simulink model "Aero_VarVsp"  (R2016b)
settings: Solver=VariableStepAuto  StartTime=0.0  StopTime=10.0  RelTol=1e-3
undefined symbols (not defined in the file or in its folder): AC
libraries: OpenFlightUtilLib x3
settings Model: Creator=UAVLAB  LastModifiedBy=rega0051
settings DataIOCC: ExternalInput=simIn  InitialState=simStateInit  StateSaveName=simStates  TimeSaveName=simTime  OutputSaveName=simOut  SignalLoggingName=simLog  DSMLoggingName=simData

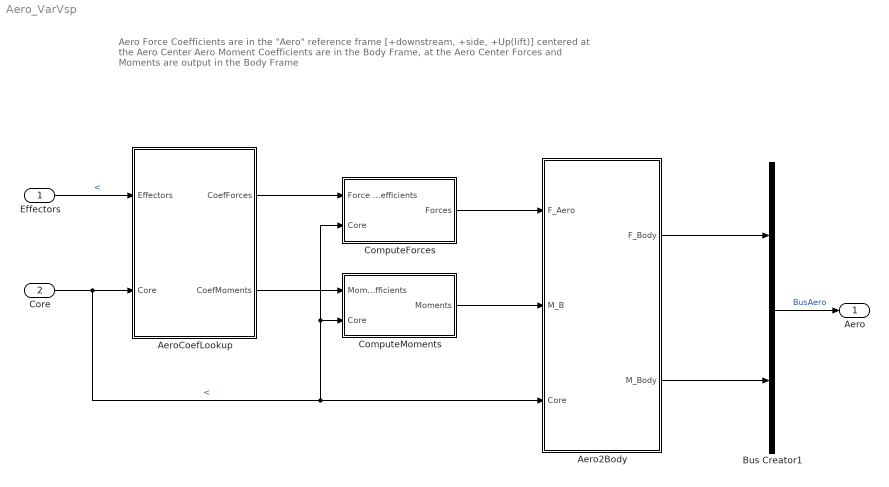
== system Aero_VarVsp ==
  note: Aero Force Coefficients are in the "Aero" reference frame [+downstream, +side, +Up(lift)] centered at the Aero Center
      | Aero Moment Coefficients are in the Body Frame, at the Aero Center
      |
      | Forces and Moments are output in the Body Frame
  Effectors : Inport  OutDataTypeStr=Bus: BusEff
  Core : Inport  Port=2  OutDataTypeStr=Bus: BusCore
  Aero2Body : Subsystem
  AeroCoefLookup : Subsystem
  Bus Creator1 : BusCreator  Inputs=2  OutDataTypeStr=Bus: BusAero
      settings: AttributesFormatString=%<OutDataTypeStr>
  ComputeForces : Subsystem
  ComputeMoments : Subsystem
  Aero : Outport  OutDataTypeStr=Bus: BusAero
  wires:
  Effectors/1 -> AeroCoefLookup/1(Effectors)  "<"
  ComputeForces/1(Forces) -> Aero2Body/1(F_Aero)
  ComputeMoments/1(Moments) -> Aero2Body/2(M_B)
  Aero2Body/1(F_Body) -> Bus Creator1/1
  Aero2Body/2(M_Body) -> Bus Creator1/2
  AeroCoefLookup/1(CoefForces) -> ComputeForces/1(Force Coefficients)
  AeroCoefLookup/2(CoefMoments) -> ComputeMoments/1(Moment Coefficients)
  Bus Creator1/1 -> Aero/1  "BusAero"
  Core/1 -> ComputeForces/2(Core), ComputeMoments/2(Core), Aero2Body/3(Core), AeroCoefLookup/2(Core)  "<"

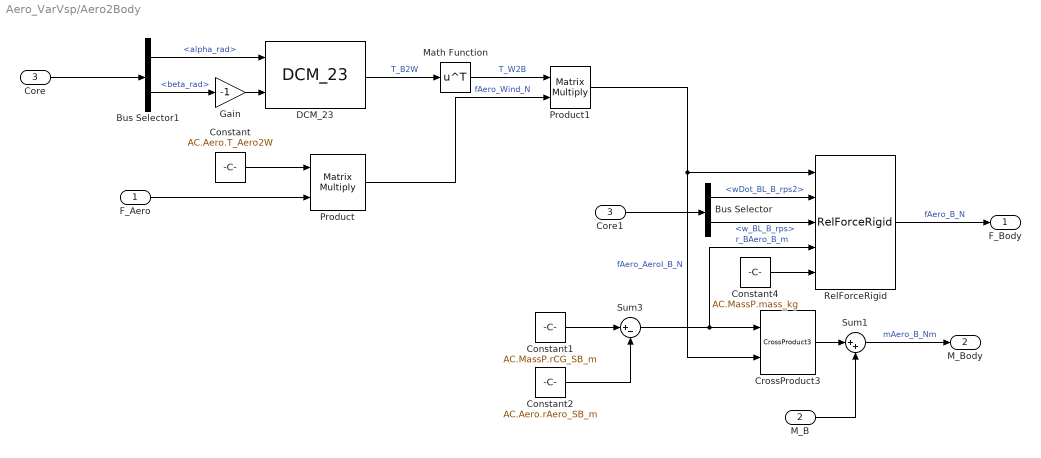
== system Aero_VarVsp/Aero2Body ==
  F_Aero : Inport
  M_B : Inport  Port=2
  Core : Inport  Port=3
  Bus Selector : BusSelector  OutputSignals=BusEom.wDot_BL_B_rps2,BusEom.w_BL_B_rps
  Bus Selector1 : BusSelector  OutputSignals=BusAux.BusFlow.alpha_rad,BusAux.BusFlow.beta_rad
  Constant : Constant  Value=AC.Aero.T_Aero2W
      settings: AttributesFormatString=%<Value>
  Constant1 : Constant  Value=AC.MassP.rCG_SB_m
      settings: AttributesFormatString=%<Value>
  Constant2 : Constant  Value=AC.Aero.rAero_SB_m
      settings: AttributesFormatString=%<Value>
  Constant4 : Constant  Value=AC.MassP.mass_kg
      settings: AttributesFormatString=%<Value>
  Core1 : InportShadow  Port=3
  CrossProduct3 : OpenFlightUtilLib/Math/CrossProduct3
  DCM_23 : OpenFlightUtilLib/Transformations/DCM_23
  Gain : Gain  Gain=-1
  Math Function : Math  Operator=transpose  SaturateOnIntegerOverflow=on
  Product : Product  Multiplication=Matrix(*)  RndMeth=Zero
  Product1 : Product  Multiplication=Matrix(*)  RndMeth=Zero
  RelForceRigid : OpenFlightUtilLib/Kinematics and Dynamics/RelForceRigid
  Sum1 : Sum  Inputs=|++  SaturateOnIntegerOverflow=on
  Sum3 : Sum  Inputs=|+-  SaturateOnIntegerOverflow=on
  F_Body : Outport
  M_Body : Outport  Port=2
  wires:
  Constant1/1 -> Sum3/1
  Constant2/1 -> Sum3/2
  Bus Selector/1 -> RelForceRigid/2  "<wDot_BL_B_rps2>"
  Bus Selector/2 -> RelForceRigid/3  "<w_BL_B_rps>"
  F_Aero/1 -> Product/2
  Constant/1 -> Product/1
  Core/1 -> Bus Selector1/1
  Math Function/1 -> Product1/1  "T_W2B"
  DCM_23/1 -> Math Function/1  "T_B2W"
  Product/1 -> Product1/2  "fAero_Wind_N"
  Product1/1 -> CrossProduct3/2, RelForceRigid/1  "fAero_AeroI_B_N"
  Sum3/1 -> RelForceRigid/4, CrossProduct3/1  "r_BAero_B_m"
  Core1/1 -> Bus Selector/1
  RelForceRigid/1 -> F_Body/1  "fAero_B_N"
  M_B/1 -> Sum1/2
  CrossProduct3/1 -> Sum1/1
  Sum1/1 -> M_Body/1  "mAero_B_Nm"
  Constant4/1 -> RelForceRigid/5
  Bus Selector1/1 -> DCM_23/1  "<alpha_rad>"
  Bus Selector1/2 -> Gain/1  "<beta_rad>"
  Gain/1 -> DCM_23/2

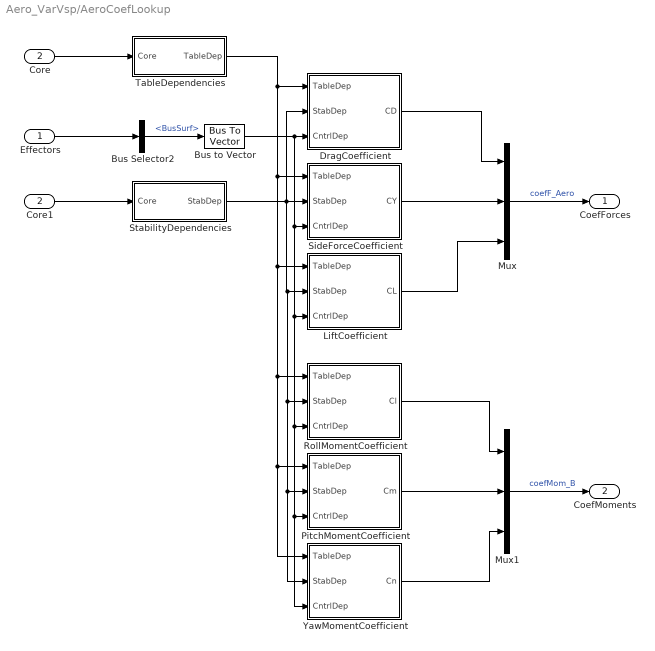
== system Aero_VarVsp/AeroCoefLookup ==
  Effectors : Inport
  Core : Inport  Port=2
  Bus Selector2 : BusSelector  OutputSignals=BusSurf
  Bus to Vector : BusToVector
  Core1 : InportShadow  Port=2
  DragCoefficient : Subsystem
  LiftCoefficient : Subsystem
  Mux : Mux  Inputs=3
  Mux1 : Mux  Inputs=3
  PitchMomentCoefficient : Subsystem
  RollMomentCoefficient : Subsystem
  SideForceCoefficient : Subsystem
  StabilityDependencies : Subsystem
  TableDependencies : Subsystem
  YawMomentCoefficient : Subsystem
  CoefForces : Outport
  CoefMoments : Outport  Port=2
  wires:
  Mux1/1 -> CoefMoments/1  "coefMom_B"
  SideForceCoefficient/1(CY) -> Mux/2
  PitchMomentCoefficient/1(Cm) -> Mux1/2
  Mux/1 -> CoefForces/1  "coefF_Aero"
  RollMomentCoefficient/1(Cl) -> Mux1/1
  LiftCoefficient/1(CL) -> Mux/3
  YawMomentCoefficient/1(Cn) -> Mux1/3
  DragCoefficient/1(CD) -> Mux/1
  Bus Selector2/1 -> Bus to Vector/1  "<BusSurf>"
  TableDependencies/1(TableDep) -> DragCoefficient/1(TableDep), SideForceCoefficient/1(TableDep), YawMomentCoefficient/1(TableDep), PitchMomentCoefficient/1(TableDep), RollMomentCoefficient/1(TableDep), LiftCoefficient/1(TableDep)
  Effectors/1 -> Bus Selector2/1
  Core1/1 -> StabilityDependencies/1(Core)
  StabilityDependencies/1(StabDep) -> DragCoefficient/2(StabDep), YawMomentCoefficient/2(StabDep), PitchMomentCoefficient/2(StabDep), RollMomentCoefficient/2(StabDep), LiftCoefficient/2(StabDep), SideForceCoefficient/2(StabDep)
  Bus to Vector/1 -> DragCoefficient/3(CntrlDep), YawMomentCoefficient/3(CntrlDep), PitchMomentCoefficient/3(CntrlDep), RollMomentCoefficient/3(CntrlDep), LiftCoefficient/3(CntrlDep), SideForceCoefficient/3(CntrlDep)
  Core/1 -> TableDependencies/1(Core)

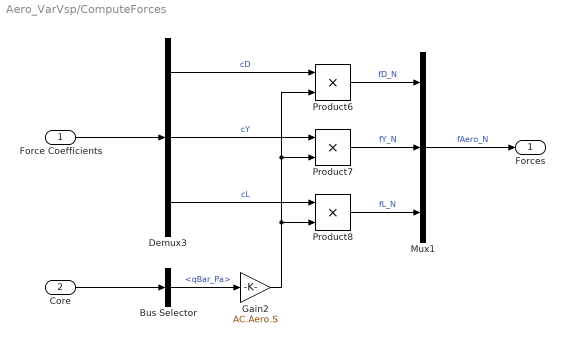
== system Aero_VarVsp/ComputeForces ==
  Force Coefficients : Inport
  Core : Inport  Port=2
  Bus Selector : BusSelector  OutputSignals=BusAux.BusFlow.qBar_Pa
  Demux3 : Demux  Outputs=3
  Gain2 : Gain  Gain=AC.Aero.S  SaturateOnIntegerOverflow=on  OutDataTypeStr=Inherit: Same as input  ParamDataTypeStr=Inherit: Same as input
      settings: AttributesFormatString=%<Gain>
  Mux1 : Mux  Inputs=3
  Product6 : Product  SaturateOnIntegerOverflow=on  InputSameDT=on  OutDataTypeStr=Inherit: Same as first input
  Product7 : Product  SaturateOnIntegerOverflow=on  InputSameDT=on  OutDataTypeStr=Inherit: Same as first input
  Product8 : Product  SaturateOnIntegerOverflow=on  InputSameDT=on  OutDataTypeStr=Inherit: Same as first input
  Forces : Outport
  wires:
  Product6/1 -> Mux1/1  "fD_N"
  Product8/1 -> Mux1/3  "fL_N"
  Product7/1 -> Mux1/2  "fY_N"
  Mux1/1 -> Forces/1  "fAero_N"
  Demux3/2 -> Product7/1  "cY"
  Demux3/1 -> Product6/1  "cD"
  Demux3/3 -> Product8/1  "cL"
  Force Coefficients/1 -> Demux3/1
  Gain2/1 -> Product6/2, Product7/2, Product8/2
  Bus Selector/1 -> Gain2/1  "<qBar_Pa>"
  Core/1 -> Bus Selector/1

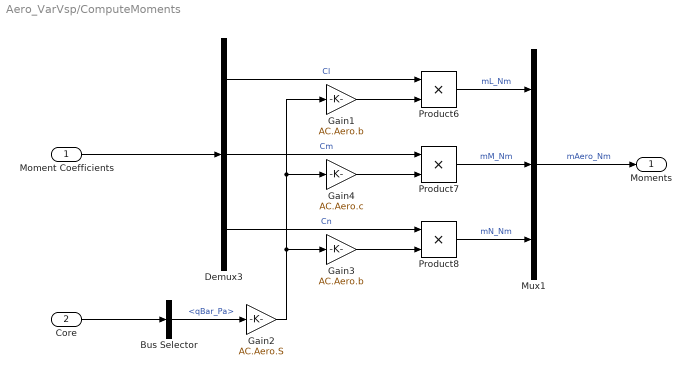
== system Aero_VarVsp/ComputeMoments ==
  Moment Coefficients : Inport
  Core : Inport  Port=2
  Bus Selector : BusSelector  OutputSignals=BusAux.BusFlow.qBar_Pa
  Demux3 : Demux  Outputs=3
  Gain1 : Gain  Gain=AC.Aero.b  SaturateOnIntegerOverflow=on  OutDataTypeStr=Inherit: Same as input  ParamDataTypeStr=Inherit: Same as input
      settings: AttributesFormatString=%<Gain>
  Gain2 : Gain  Gain=AC.Aero.S  SaturateOnIntegerOverflow=on  OutDataTypeStr=Inherit: Same as input  ParamDataTypeStr=Inherit: Same as input
      settings: AttributesFormatString=%<Gain>
  Gain3 : Gain  Gain=AC.Aero.b  SaturateOnIntegerOverflow=on  OutDataTypeStr=Inherit: Same as input  ParamDataTypeStr=Inherit: Same as input
      settings: AttributesFormatString=%<Gain>
  Gain4 : Gain  Gain=AC.Aero.c  SaturateOnIntegerOverflow=on  OutDataTypeStr=Inherit: Same as input  ParamDataTypeStr=Inherit: Same as input
      settings: AttributesFormatString=%<Gain>
  Mux1 : Mux  Inputs=3
  Product6 : Product  SaturateOnIntegerOverflow=on  InputSameDT=on  OutDataTypeStr=Inherit: Same as first input
  Product7 : Product  SaturateOnIntegerOverflow=on  InputSameDT=on  OutDataTypeStr=Inherit: Same as first input
  Product8 : Product  SaturateOnIntegerOverflow=on  InputSameDT=on  OutDataTypeStr=Inherit: Same as first input
  Moments : Outport
  wires:
  Product6/1 -> Mux1/1  "mL_Nm"
  Product8/1 -> Mux1/3  "mN_Nm"
  Moment Coefficients/1 -> Demux3/1
  Product7/1 -> Mux1/2  "mM_Nm"
  Gain3/1 -> Product8/2
  Mux1/1 -> Moments/1  "mAero_Nm"
  Gain1/1 -> Product6/2
  Gain2/1 -> Gain1/1, Gain4/1, Gain3/1
  Demux3/2 -> Product7/1  "Cm"
  Gain4/1 -> Product7/2
  Demux3/1 -> Product6/1  "Cl"
  Demux3/3 -> Product8/1  "Cn"
  Bus Selector/1 -> Gain2/1  "<qBar_Pa>"
  Core/1 -> Bus Selector/1

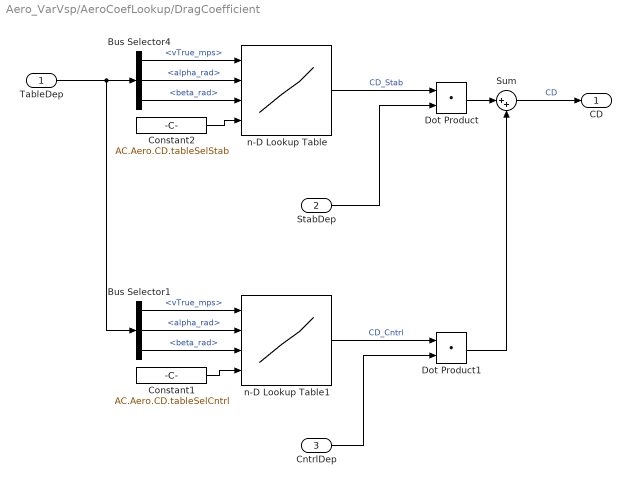
== system Aero_VarVsp/AeroCoefLookup/DragCoefficient ==
  TableDep : Inport
  StabDep : Inport  Port=2
  CntrlDep : Inport  Port=3
  Bus Selector1 : BusSelector  OutputSignals=vTrue_mps,alpha_rad,beta_rad
  Bus Selector4 : BusSelector  OutputSignals=vTrue_mps,alpha_rad,beta_rad
  Constant1 : Constant  Value=AC.Aero.CD.tableSelCntrl
      settings: AttributesFormatString=%<Value>
  Constant2 : Constant  Value=AC.Aero.CD.tableSelStab
      settings: AttributesFormatString=%<Value>
  Dot Product : DotProduct  InputSameDT=on  OutDataTypeStr=Inherit: Inherit via internal rule
  Dot Product1 : DotProduct  InputSameDT=on  OutDataTypeStr=Inherit: Inherit via internal rule
  Sum : Sum  Inputs=|++
  n-D Lookup Table : Lookup_n-D  NumberOfTableDimensions=AC.Aero.tableDim  BreakpointsForDimension1=AC.Aero.breakPts{1}  BreakpointsForDimension2=AC.Aero.breakPts{2}  BreakpointsForDimension3=AC.Aero.breakPts{3}  BreakpointsForDimension4=AC.Aero.CD.tableSelStab  Table=AC.Aero.CD.tableStab  InternalRulePriority=Speed  RndMeth=Simplest  InputSameDT=on
      settings: AttributesFormatString=%<Table>
  n-D Lookup Table1 : Lookup_n-D  NumberOfTableDimensions=AC.Aero.tableDim  BreakpointsForDimension1=AC.Aero.breakPts{1}  BreakpointsForDimension2=AC.Aero.breakPts{2}  BreakpointsForDimension3=AC.Aero.breakPts{3}  BreakpointsForDimension4=AC.Aero.CD.tableSelCntrl  Table=AC.Aero.CD.tableCntrl  InternalRulePriority=Speed  RndMeth=Simplest  InputSameDT=on
      settings: AttributesFormatString=%<Table>
  CD : Outport
  wires:
  Dot Product/1 -> Sum/1
  Bus Selector4/1 -> n-D Lookup Table/1  "<vTrue_mps>"
  Bus Selector4/2 -> n-D Lookup Table/2  "<alpha_rad>"
  Constant2/1 -> n-D Lookup Table/4
  n-D Lookup Table/1 -> Dot Product/1  "CD_Stab"
  StabDep/1 -> Dot Product/2
  TableDep/1 -> Bus Selector1/1, Bus Selector4/1
  Constant1/1 -> n-D Lookup Table1/4
  CntrlDep/1 -> Dot Product1/2
  n-D Lookup Table1/1 -> Dot Product1/1  "CD_Cntrl"
  Dot Product1/1 -> Sum/2
  Sum/1 -> CD/1  "CD"
  Bus Selector4/3 -> n-D Lookup Table/3  "<beta_rad>"
  Bus Selector1/1 -> n-D Lookup Table1/1  "<vTrue_mps>"
  Bus Selector1/2 -> n-D Lookup Table1/2  "<alpha_rad>"
  Bus Selector1/3 -> n-D Lookup Table1/3  "<beta_rad>"

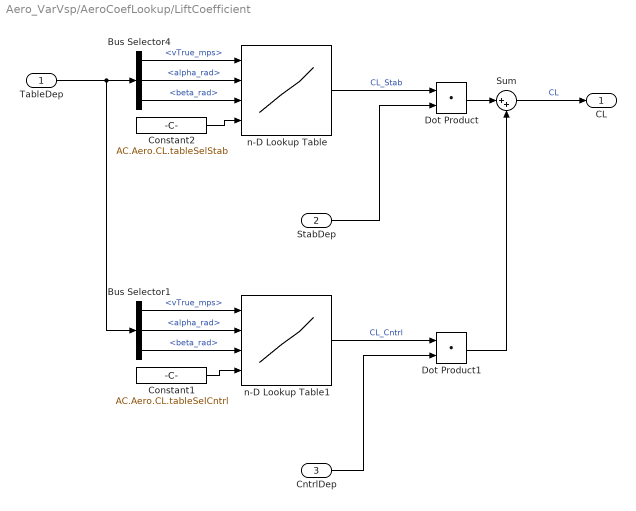
== system Aero_VarVsp/AeroCoefLookup/LiftCoefficient ==
  TableDep : Inport
  StabDep : Inport  Port=2
  CntrlDep : Inport  Port=3
  Bus Selector1 : BusSelector  OutputSignals=vTrue_mps,alpha_rad,beta_rad
  Bus Selector4 : BusSelector  OutputSignals=vTrue_mps,alpha_rad,beta_rad
  Constant1 : Constant  Value=AC.Aero.CL.tableSelCntrl
      settings: AttributesFormatString=%<Value>
  Constant2 : Constant  Value=AC.Aero.CL.tableSelStab
      settings: AttributesFormatString=%<Value>
  Dot Product : DotProduct  InputSameDT=on  OutDataTypeStr=Inherit: Inherit via internal rule
  Dot Product1 : DotProduct  InputSameDT=on  OutDataTypeStr=Inherit: Inherit via internal rule
  Sum : Sum  Inputs=|++
  n-D Lookup Table : Lookup_n-D  NumberOfTableDimensions=AC.Aero.tableDim  BreakpointsForDimension1=AC.Aero.breakPts{1}  BreakpointsForDimension2=AC.Aero.breakPts{2}  BreakpointsForDimension3=AC.Aero.breakPts{3}  BreakpointsForDimension4=AC.Aero.CL.tableSelStab  Table=AC.Aero.CL.tableStab  InternalRulePriority=Speed  RndMeth=Simplest  InputSameDT=on
      settings: AttributesFormatString=%<Table>
  n-D Lookup Table1 : Lookup_n-D  NumberOfTableDimensions=AC.Aero.tableDim  BreakpointsForDimension1=AC.Aero.breakPts{1}  BreakpointsForDimension2=AC.Aero.breakPts{2}  BreakpointsForDimension3=AC.Aero.breakPts{3}  BreakpointsForDimension4=AC.Aero.CL.tableSelCntrl  Table=AC.Aero.CL.tableCntrl  InternalRulePriority=Speed  RndMeth=Simplest  InputSameDT=on
      settings: AttributesFormatString=%<Table>
  CL : Outport
  wires:
  Dot Product/1 -> Sum/1
  Constant2/1 -> n-D Lookup Table/4
  n-D Lookup Table/1 -> Dot Product/1  "CL_Stab"
  StabDep/1 -> Dot Product/2
  TableDep/1 -> Bus Selector1/1, Bus Selector4/1
  Constant1/1 -> n-D Lookup Table1/4
  CntrlDep/1 -> Dot Product1/2
  n-D Lookup Table1/1 -> Dot Product1/1  "CL_Cntrl"
  Dot Product1/1 -> Sum/2
  Sum/1 -> CL/1  "CL"
  Bus Selector4/3 -> n-D Lookup Table/3  "<beta_rad>"
  Bus Selector4/2 -> n-D Lookup Table/2  "<alpha_rad>"
  Bus Selector4/1 -> n-D Lookup Table/1  "<vTrue_mps>"
  Bus Selector1/1 -> n-D Lookup Table1/1  "<vTrue_mps>"
  Bus Selector1/2 -> n-D Lookup Table1/2  "<alpha_rad>"
  Bus Selector1/3 -> n-D Lookup Table1/3  "<beta_rad>"

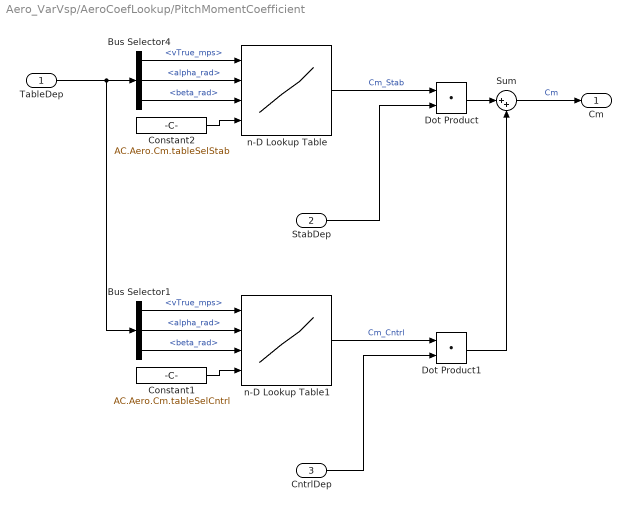
== system Aero_VarVsp/AeroCoefLookup/PitchMomentCoefficient ==
  TableDep : Inport
  StabDep : Inport  Port=2
  CntrlDep : Inport  Port=3
  Bus Selector1 : BusSelector  OutputSignals=vTrue_mps,alpha_rad,beta_rad
  Bus Selector4 : BusSelector  OutputSignals=vTrue_mps,alpha_rad,beta_rad
  Constant1 : Constant  Value=AC.Aero.Cm.tableSelCntrl
      settings: AttributesFormatString=%<Value>
  Constant2 : Constant  Value=AC.Aero.Cm.tableSelStab
      settings: AttributesFormatString=%<Value>
  Dot Product : DotProduct  InputSameDT=on  OutDataTypeStr=Inherit: Inherit via internal rule
  Dot Product1 : DotProduct  InputSameDT=on  OutDataTypeStr=Inherit: Inherit via internal rule
  Sum : Sum  Inputs=|++
  n-D Lookup Table : Lookup_n-D  NumberOfTableDimensions=AC.Aero.tableDim  BreakpointsForDimension1=AC.Aero.breakPts{1}  BreakpointsForDimension2=AC.Aero.breakPts{2}  BreakpointsForDimension3=AC.Aero.breakPts{3}  BreakpointsForDimension4=AC.Aero.Cm.tableSelStab  Table=AC.Aero.Cm.tableStab  InternalRulePriority=Speed  RndMeth=Simplest  InputSameDT=on
      settings: AttributesFormatString=%<Table>
  n-D Lookup Table1 : Lookup_n-D  NumberOfTableDimensions=AC.Aero.tableDim  BreakpointsForDimension1=AC.Aero.breakPts{1}  BreakpointsForDimension2=AC.Aero.breakPts{2}  BreakpointsForDimension3=AC.Aero.breakPts{3}  BreakpointsForDimension4=AC.Aero.Cm.tableSelCntrl  Table=AC.Aero.Cm.tableCntrl  InternalRulePriority=Speed  RndMeth=Simplest  InputSameDT=on
      settings: AttributesFormatString=%<Table>
  Cm : Outport
  wires:
  Dot Product/1 -> Sum/1
  Constant2/1 -> n-D Lookup Table/4
  n-D Lookup Table/1 -> Dot Product/1  "Cm_Stab"
  StabDep/1 -> Dot Product/2
  TableDep/1 -> Bus Selector1/1, Bus Selector4/1
  Constant1/1 -> n-D Lookup Table1/4
  CntrlDep/1 -> Dot Product1/2
  n-D Lookup Table1/1 -> Dot Product1/1  "Cm_Cntrl"
  Dot Product1/1 -> Sum/2
  Sum/1 -> Cm/1  "Cm"
  Bus Selector1/1 -> n-D Lookup Table1/1  "<vTrue_mps>"
  Bus Selector1/3 -> n-D Lookup Table1/3  "<beta_rad>"
  Bus Selector1/2 -> n-D Lookup Table1/2  "<alpha_rad>"
  Bus Selector4/3 -> n-D Lookup Table/3  "<beta_rad>"
  Bus Selector4/2 -> n-D Lookup Table/2  "<alpha_rad>"
  Bus Selector4/1 -> n-D Lookup Table/1  "<vTrue_mps>"

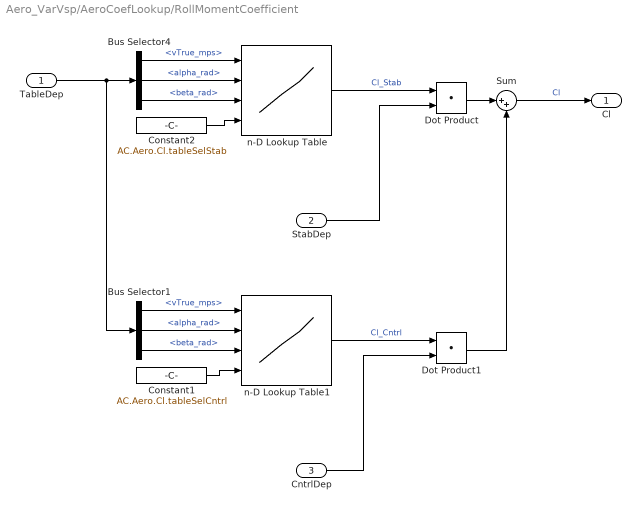
== system Aero_VarVsp/AeroCoefLookup/RollMomentCoefficient ==
  TableDep : Inport
  StabDep : Inport  Port=2
  CntrlDep : Inport  Port=3
  Bus Selector1 : BusSelector  OutputSignals=vTrue_mps,alpha_rad,beta_rad
  Bus Selector4 : BusSelector  OutputSignals=vTrue_mps,alpha_rad,beta_rad
  Constant1 : Constant  Value=AC.Aero.Cl.tableSelCntrl
      settings: AttributesFormatString=%<Value>
  Constant2 : Constant  Value=AC.Aero.Cl.tableSelStab
      settings: AttributesFormatString=%<Value>
  Dot Product : DotProduct  InputSameDT=on  OutDataTypeStr=Inherit: Inherit via internal rule
  Dot Product1 : DotProduct  InputSameDT=on  OutDataTypeStr=Inherit: Inherit via internal rule
  Sum : Sum  Inputs=|++
  n-D Lookup Table : Lookup_n-D  NumberOfTableDimensions=AC.Aero.tableDim  BreakpointsForDimension1=AC.Aero.breakPts{1}  BreakpointsForDimension2=AC.Aero.breakPts{2}  BreakpointsForDimension3=AC.Aero.breakPts{3}  BreakpointsForDimension4=AC.Aero.Cl.tableSelStab  Table=AC.Aero.Cl.tableStab  InternalRulePriority=Speed  RndMeth=Simplest  InputSameDT=on
      settings: AttributesFormatString=%<Table>
  n-D Lookup Table1 : Lookup_n-D  NumberOfTableDimensions=AC.Aero.tableDim  BreakpointsForDimension1=AC.Aero.breakPts{1}  BreakpointsForDimension2=AC.Aero.breakPts{2}  BreakpointsForDimension3=AC.Aero.breakPts{3}  BreakpointsForDimension4=AC.Aero.Cl.tableSelCntrl  Table=AC.Aero.Cl.tableCntrl  InternalRulePriority=Speed  RndMeth=Simplest  InputSameDT=on
      settings: AttributesFormatString=%<Table>
  Cl : Outport
  wires:
  Dot Product/1 -> Sum/1
  Constant2/1 -> n-D Lookup Table/4
  n-D Lookup Table/1 -> Dot Product/1  "Cl_Stab"
  StabDep/1 -> Dot Product/2
  TableDep/1 -> Bus Selector1/1, Bus Selector4/1
  Constant1/1 -> n-D Lookup Table1/4
  CntrlDep/1 -> Dot Product1/2
  n-D Lookup Table1/1 -> Dot Product1/1  "Cl_Cntrl"
  Dot Product1/1 -> Sum/2
  Sum/1 -> Cl/1  "Cl"
  Bus Selector4/1 -> n-D Lookup Table/1  "<vTrue_mps>"
  Bus Selector4/2 -> n-D Lookup Table/2  "<alpha_rad>"
  Bus Selector4/3 -> n-D Lookup Table/3  "<beta_rad>"
  Bus Selector1/1 -> n-D Lookup Table1/1  "<vTrue_mps>"
  Bus Selector1/2 -> n-D Lookup Table1/2  "<alpha_rad>"
  Bus Selector1/3 -> n-D Lookup Table1/3  "<beta_rad>"

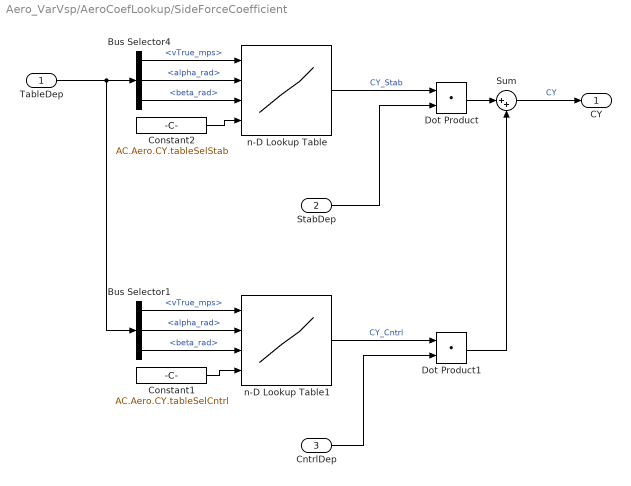
== system Aero_VarVsp/AeroCoefLookup/SideForceCoefficient ==
  TableDep : Inport
  StabDep : Inport  Port=2
  CntrlDep : Inport  Port=3
  Bus Selector1 : BusSelector  OutputSignals=vTrue_mps,alpha_rad,beta_rad
  Bus Selector4 : BusSelector  OutputSignals=vTrue_mps,alpha_rad,beta_rad
  Constant1 : Constant  Value=AC.Aero.CY.tableSelCntrl
      settings: AttributesFormatString=%<Value>
  Constant2 : Constant  Value=AC.Aero.CY.tableSelStab
      settings: AttributesFormatString=%<Value>
  Dot Product : DotProduct  InputSameDT=on  OutDataTypeStr=Inherit: Inherit via internal rule
  Dot Product1 : DotProduct  InputSameDT=on  OutDataTypeStr=Inherit: Inherit via internal rule
  Sum : Sum  Inputs=|++
  n-D Lookup Table : Lookup_n-D  NumberOfTableDimensions=AC.Aero.tableDim  BreakpointsForDimension1=AC.Aero.breakPts{1}  BreakpointsForDimension2=AC.Aero.breakPts{2}  BreakpointsForDimension3=AC.Aero.breakPts{3}  BreakpointsForDimension4=AC.Aero.CY.tableSelStab  Table=AC.Aero.CY.tableStab  InternalRulePriority=Speed  RndMeth=Simplest  InputSameDT=on
      settings: AttributesFormatString=%<Table>
  n-D Lookup Table1 : Lookup_n-D  NumberOfTableDimensions=AC.Aero.tableDim  BreakpointsForDimension1=AC.Aero.breakPts{1}  BreakpointsForDimension2=AC.Aero.breakPts{2}  BreakpointsForDimension3=AC.Aero.breakPts{3}  BreakpointsForDimension4=AC.Aero.CY.tableSelCntrl  Table=AC.Aero.CY.tableCntrl  InternalRulePriority=Speed  RndMeth=Simplest  InputSameDT=on
      settings: AttributesFormatString=%<Table>
  CY : Outport
  wires:
  Dot Product/1 -> Sum/1
  Bus Selector4/1 -> n-D Lookup Table/1  "<vTrue_mps>"
  Bus Selector4/2 -> n-D Lookup Table/2  "<alpha_rad>"
  Constant2/1 -> n-D Lookup Table/4
  n-D Lookup Table/1 -> Dot Product/1  "CY_Stab"
  StabDep/1 -> Dot Product/2
  TableDep/1 -> Bus Selector1/1, Bus Selector4/1
  Constant1/1 -> n-D Lookup Table1/4
  CntrlDep/1 -> Dot Product1/2
  n-D Lookup Table1/1 -> Dot Product1/1  "CY_Cntrl"
  Dot Product1/1 -> Sum/2
  Sum/1 -> CY/1  "CY"
  Bus Selector4/3 -> n-D Lookup Table/3  "<beta_rad>"
  Bus Selector1/1 -> n-D Lookup Table1/1  "<vTrue_mps>"
  Bus Selector1/2 -> n-D Lookup Table1/2  "<alpha_rad>"
  Bus Selector1/3 -> n-D Lookup Table1/3  "<beta_rad>"

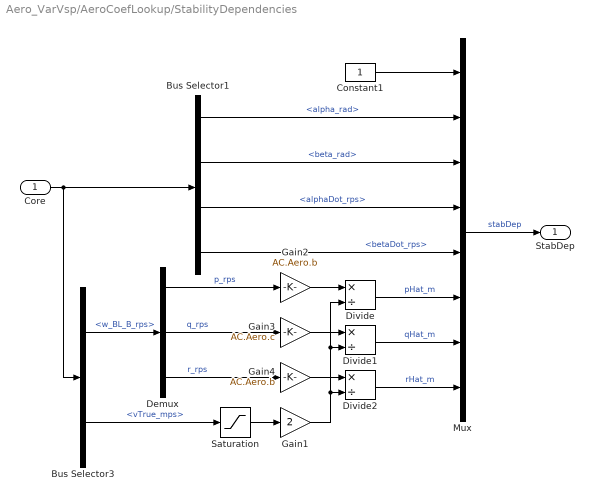
== system Aero_VarVsp/AeroCoefLookup/StabilityDependencies ==
  Core : Inport
  Bus Selector1 : BusSelector  OutputSignals=BusAux.BusFlow.alpha_rad,BusAux.BusFlow.beta_rad,BusAux.BusFlow.alphaDot_rps,BusAux.BusFlow.betaDot_rps
  Bus Selector3 : BusSelector  OutputSignals=BusEom.w_BL_B_rps,BusAux.BusFlow.vTrue_mps
  Constant1 : Constant
  Demux : Demux  Outputs=3
  Divide : Product  Inputs=*/
  Divide1 : Product  Inputs=*/
  Divide2 : Product  Inputs=*/
  Gain1 : Gain  Gain=2  SaturateOnIntegerOverflow=on  OutDataTypeStr=Inherit: Same as input  ParamDataTypeStr=Inherit: Same as input
  Gain2 : Gain  Gain=AC.Aero.b  SaturateOnIntegerOverflow=on  OutDataTypeStr=Inherit: Same as input  ParamDataTypeStr=Inherit: Same as input
      settings: AttributesFormatString=%<Gain>
  Gain3 : Gain  Gain=AC.Aero.c  SaturateOnIntegerOverflow=on  OutDataTypeStr=Inherit: Same as input  ParamDataTypeStr=Inherit: Same as input
      settings: AttributesFormatString=%<Gain>
  Gain4 : Gain  Gain=AC.Aero.b  SaturateOnIntegerOverflow=on  OutDataTypeStr=Inherit: Same as input  ParamDataTypeStr=Inherit: Same as input
      settings: AttributesFormatString=%<Gain>
  Mux : Mux  Inputs=length(AC.Aero.CL.tableSelStab)
  Saturation : Saturate  UpperLimit=inf  LowerLimit=0.1
  StabDep : Outport
  wires:
  Bus Selector1/3 -> Mux/4  "<alphaDot_rps>"
  Divide/1 -> Mux/6  "pHat_m"
  Bus Selector1/2 -> Mux/3  "<beta_rad>"
  Bus Selector1/4 -> Mux/5  "<betaDot_rps>"
  Core/1 -> Bus Selector3/1, Bus Selector1/1
  Constant1/1 -> Mux/1
  Mux/1 -> StabDep/1  "stabDep"
  Bus Selector1/1 -> Mux/2  "<alpha_rad>"
  Gain2/1 -> Divide/1
  Gain1/1 -> Divide1/2, Divide/2, Divide2/2
  Divide1/1 -> Mux/7  "qHat_m"
  Divide2/1 -> Mux/8  "rHat_m"
  Gain3/1 -> Divide1/1
  Gain4/1 -> Divide2/1
  Bus Selector3/2 -> Saturation/1  "<vTrue_mps>"
  Saturation/1 -> Gain1/1
  Bus Selector3/1 -> Demux/1  "<w_BL_B_rps>"
  Demux/1 -> Gain2/1  "p_rps"
  Demux/2 -> Gain3/1  "q_rps"
  Demux/3 -> Gain4/1  "r_rps"

== system Aero_VarVsp/AeroCoefLookup/TableDependencies ==
  Core : Inport
  Bus Creator : BusCreator  Inputs=3
  Bus Selector4 : BusSelector  OutputSignals=BusAux.BusFlow.vTrue_mps,BusAux.BusFlow.alpha_rad,BusAux.BusFlow.beta_rad
  TableDep : Outport
  wires:
  Core/1 -> Bus Selector4/1
  Bus Selector4/1 -> Bus Creator/1  "<vTrue_mps>"
  Bus Selector4/3 -> Bus Creator/3  "<beta_rad>"
  Bus Selector4/2 -> Bus Creator/2  "<alpha_rad>"
  Bus Creator/1 -> TableDep/1  "tableDep"

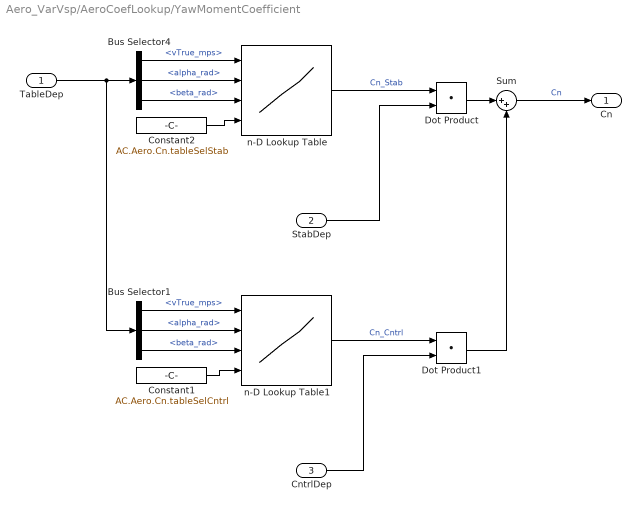
== system Aero_VarVsp/AeroCoefLookup/YawMomentCoefficient ==
  TableDep : Inport
  StabDep : Inport  Port=2
  CntrlDep : Inport  Port=3
  Bus Selector1 : BusSelector  OutputSignals=vTrue_mps,alpha_rad,beta_rad
  Bus Selector4 : BusSelector  OutputSignals=vTrue_mps,alpha_rad,beta_rad
  Constant1 : Constant  Value=AC.Aero.Cn.tableSelCntrl
      settings: AttributesFormatString=%<Value>
  Constant2 : Constant  Value=AC.Aero.Cn.tableSelStab
      settings: AttributesFormatString=%<Value>
  Dot Product : DotProduct  InputSameDT=on  OutDataTypeStr=Inherit: Inherit via internal rule
  Dot Product1 : DotProduct  InputSameDT=on  OutDataTypeStr=Inherit: Inherit via internal rule
  Sum : Sum  Inputs=|++
  n-D Lookup Table : Lookup_n-D  NumberOfTableDimensions=AC.Aero.tableDim  BreakpointsForDimension1=AC.Aero.breakPts{1}  BreakpointsForDimension2=AC.Aero.breakPts{2}  BreakpointsForDimension3=AC.Aero.breakPts{3}  BreakpointsForDimension4=AC.Aero.Cn.tableSelStab  Table=AC.Aero.Cn.tableStab  InternalRulePriority=Speed  RndMeth=Simplest  InputSameDT=on
      settings: AttributesFormatString=%<Table>
  n-D Lookup Table1 : Lookup_n-D  NumberOfTableDimensions=AC.Aero.tableDim  BreakpointsForDimension1=AC.Aero.breakPts{1}  BreakpointsForDimension2=AC.Aero.breakPts{2}  BreakpointsForDimension3=AC.Aero.breakPts{3}  BreakpointsForDimension4=AC.Aero.Cn.tableSelCntrl  Table=AC.Aero.Cn.tableCntrl  InternalRulePriority=Speed  RndMeth=Simplest  InputSameDT=on
      settings: AttributesFormatString=%<Table>
  Cn : Outport
  wires:
  Dot Product/1 -> Sum/1
  Constant2/1 -> n-D Lookup Table/4
  n-D Lookup Table/1 -> Dot Product/1  "Cn_Stab"
  StabDep/1 -> Dot Product/2
  TableDep/1 -> Bus Selector1/1, Bus Selector4/1
  Constant1/1 -> n-D Lookup Table1/4
  CntrlDep/1 -> Dot Product1/2
  n-D Lookup Table1/1 -> Dot Product1/1  "Cn_Cntrl"
  Dot Product1/1 -> Sum/2
  Sum/1 -> Cn/1  "Cn"
  Bus Selector1/1 -> n-D Lookup Table1/1  "<vTrue_mps>"
  Bus Selector1/2 -> n-D Lookup Table1/2  "<alpha_rad>"
  Bus Selector1/3 -> n-D Lookup Table1/3  "<beta_rad>"
  Bus Selector4/1 -> n-D Lookup Table/1  "<vTrue_mps>"
  Bus Selector4/2 -> n-D Lookup Table/2  "<alpha_rad>"
  Bus Selector4/3 -> n-D Lookup Table/3  "<beta_rad>"
